simulink model "P_PDsim"  (R2018b)
settings: Solver=VariableStepAuto  StartTime=0.0  StopTime=70  RelTol=1e-3
values from neighbouring files (symbols this model uses):
  C = (pi*(100*10^-3)^2)/4    (= 0.00785398163397)    [Siviseviyesistemkodu.m]
  h = 0.225    [Siviseviyesistemkodu.m]
  P = 7.08    [Siviseviyesistemkodu.m]
  qin = 0.000087083333    (= 8.7083333e-05)    [Siviseviyesistemkodu.m]
  R = (h)/qo    [Siviseviyesistemkodu.m]
  td = 0.56    [Siviseviyesistemkodu.m]
settings Model: Creator=Yasin  LastModifiedBy=Yasin

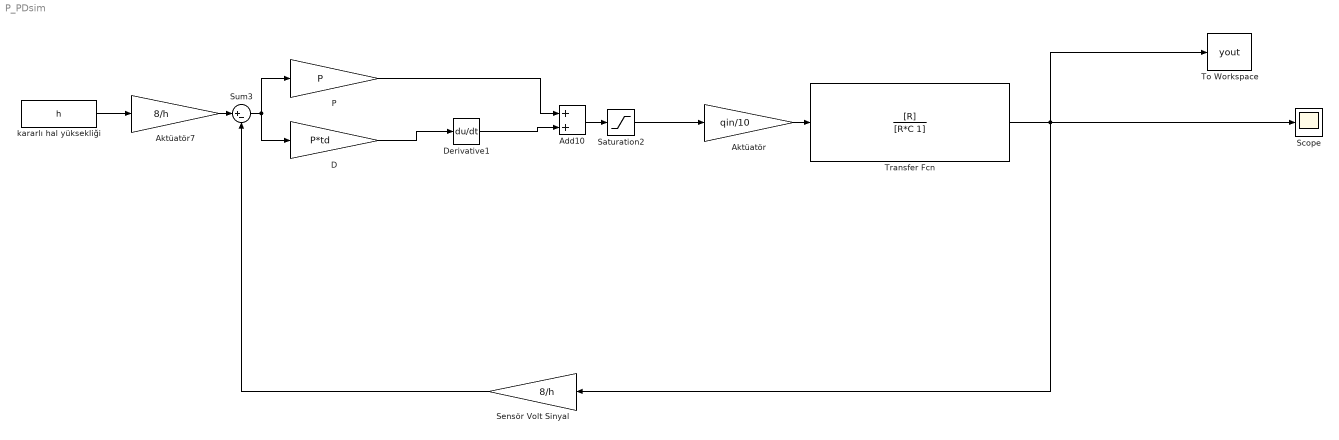
== system P_PDsim ==
  Add10 : Sum
  Aktüatör : Gain  Gain=qin/10
  Aktüatör7 : Gain  Gain=8/h
  D : Gain  Gain=P*td
  Derivative1 : Derivative
  P : Gain  Gain=P
  Saturation2 : Saturate  UpperLimit=10  LowerLimit=0  ZeroCross=off
  Scope : Scope
  Sensör Volt Sinyal : Gain  Gain=8/h
  Sum3 : Sum  Inputs=|+-
  To Workspace : ToWorkspace  VariableName=yout  SaveFormat=Structure With Time  SampleTime=-1
      settings: Save2DSignal=2-D array (concatenate along first dimension)
  Transfer Fcn : TransferFcn  Numerator=[R]  Denominator=[R*C 1]
  kararlı hal yüksekliği : Constant  Value=h
  wires:
  Sensör Volt Sinyal/1 -> Sum3/2
  kararlı hal yüksekliği/1 -> Aktüatör7/1
  Aktüatör/1 -> Transfer Fcn/1
  Add10/1 -> Saturation2/1
  P/1 -> Add10/1
  Aktüatör7/1 -> Sum3/1
  Saturation2/1 -> Aktüatör/1
  Sum3/1 -> D/1, P/1
  D/1 -> Derivative1/1
  Transfer Fcn/1 -> To Workspace/1, Scope/1, Sensör Volt Sinyal/1
  Derivative1/1 -> Add10/2
